simulink model "cpu_von_nuemann"  (R2020a)
settings: Solver=VariableStepAuto  StartTime=0.0  StopTime=10.0  RelTol=1e-3
libraries: simulink_extras x402, msbPllFoundation x1
(part 16 of 64)

== system cpu_von_nuemann/CPU/ALU/Subsystem7/Subsystem1/Subsystem4/Subsystem1 ==
  In1 : Inport
  In2 : Inport  Port=2
  In3 : Inport  Port=3
  In4 : Inport  Port=4
  In5 : Inport  Port=5
  In6 : Inport  Port=6
  In7 : Inport  Port=7
  NAND : Logic  Operator=NAND  AllPortsSameDT=off  OutDataTypeStr=boolean
  NAND{1..2,4..6} (5 alike) : Logic  Operator=NAND  Inputs=4  AllPortsSameDT=off  OutDataTypeStr=boolean
  NAND3 : Logic  Operator=NAND  AllPortsSameDT=off  OutDataTypeStr=boolean
  Out1 : Outport
  wires:
  NAND6/1 -> NAND1/4
  In5/1 -> NAND5/3
  NAND3/1 -> NAND4/2, NAND2/2
  In1/1 -> NAND6/2, NAND5/2, NAND3/2, NAND3/1
  In2/1 -> NAND6/1, NAND4/1, NAND/2, NAND/1
  In4/1 -> NAND4/3
  In3/1 -> NAND2/3
  NAND/1 -> NAND5/1, NAND2/1
  NAND1/1 -> Out1/1
  In6/1 -> NAND6/3
  NAND5/1 -> NAND1/3
  NAND4/1 -> NAND1/2
  In7/1 -> NAND2/4, NAND4/4, NAND5/4, NAND6/4
  NAND2/1 -> NAND1/1

== system cpu_von_nuemann/CPU/ALU/Subsystem7/Subsystem1/Subsystem4/Subsystem2 ==
  In1 : Inport
  In2 : Inport  Port=2
  In3 : Inport  Port=3
  In4 : Inport  Port=4
  In5 : Inport  Port=5
  In6 : Inport  Port=6
  In7 : Inport  Port=7
  NAND : Logic  Operator=NAND  AllPortsSameDT=off  OutDataTypeStr=boolean
  NAND{1..2,4..6} (5 alike) : Logic  Operator=NAND  Inputs=4  AllPortsSameDT=off  OutDataTypeStr=boolean
  NAND3 : Logic  Operator=NAND  AllPortsSameDT=off  OutDataTypeStr=boolean
  Out1 : Outport
  wires:
  NAND6/1 -> NAND1/4
  In5/1 -> NAND5/3
  NAND3/1 -> NAND4/2, NAND2/2
  In1/1 -> NAND6/2, NAND5/2, NAND3/2, NAND3/1
  In2/1 -> NAND6/1, NAND4/1, NAND/2, NAND/1
  In4/1 -> NAND4/3
  In3/1 -> NAND2/3
  NAND/1 -> NAND5/1, NAND2/1
  NAND1/1 -> Out1/1
  In6/1 -> NAND6/3
  NAND5/1 -> NAND1/3
  NAND4/1 -> NAND1/2
  In7/1 -> NAND2/4, NAND4/4, NAND5/4, NAND6/4
  NAND2/1 -> NAND1/1

== system cpu_von_nuemann/CPU/ALU/Subsystem7/Subsystem1/Subsystem4/Subsystem3 ==
  In1 : Inport
  In2 : Inport  Port=2
  In3 : Inport  Port=3
  In4 : Inport  Port=4
  In5 : Inport  Port=5
  In6 : Inport  Port=6
  In7 : Inport  Port=7
  NAND : Logic  Operator=NAND  AllPortsSameDT=off  OutDataTypeStr=boolean
  NAND{1..2,4..6} (5 alike) : Logic  Operator=NAND  Inputs=4  AllPortsSameDT=off  OutDataTypeStr=boolean
  NAND3 : Logic  Operator=NAND  AllPortsSameDT=off  OutDataTypeStr=boolean
  Out1 : Outport
  wires:
  NAND6/1 -> NAND1/4
  In5/1 -> NAND5/3
  NAND3/1 -> NAND4/2, NAND2/2
  In1/1 -> NAND6/2, NAND5/2, NAND3/2, NAND3/1
  In2/1 -> NAND6/1, NAND4/1, NAND/2, NAND/1
  In4/1 -> NAND4/3
  In3/1 -> NAND2/3
  NAND/1 -> NAND5/1, NAND2/1
  NAND1/1 -> Out1/1
  In6/1 -> NAND6/3
  NAND5/1 -> NAND1/3
  NAND4/1 -> NAND1/2
  In7/1 -> NAND2/4, NAND4/4, NAND5/4, NAND6/4
  NAND2/1 -> NAND1/1

== system cpu_von_nuemann/CPU/ALU/Subsystem7/Subsystem1/Subsystem4/Subsystem4 ==
  In1 : Inport
  In2 : Inport  Port=2
  In3 : Inport  Port=3
  In4 : Inport  Port=4
  In5 : Inport  Port=5
  In6 : Inport  Port=6
  In7 : Inport  Port=7
  NAND : Logic  Operator=NAND  AllPortsSameDT=off  OutDataTypeStr=boolean
  NAND{1..2,4..6} (5 alike) : Logic  Operator=NAND  Inputs=4  AllPortsSameDT=off  OutDataTypeStr=boolean
  NAND3 : Logic  Operator=NAND  AllPortsSameDT=off  OutDataTypeStr=boolean
  Out1 : Outport
  wires:
  NAND6/1 -> NAND1/4
  In5/1 -> NAND5/3
  NAND3/1 -> NAND4/2, NAND2/2
  In1/1 -> NAND6/2, NAND5/2, NAND3/2, NAND3/1
  In2/1 -> NAND6/1, NAND4/1, NAND/2, NAND/1
  In4/1 -> NAND4/3
  In3/1 -> NAND2/3
  NAND/1 -> NAND5/1, NAND2/1
  NAND1/1 -> Out1/1
  In6/1 -> NAND6/3
  NAND5/1 -> NAND1/3
  NAND4/1 -> NAND1/2
  In7/1 -> NAND2/4, NAND4/4, NAND5/4, NAND6/4
  NAND2/1 -> NAND1/1

== system cpu_von_nuemann/CPU/ALU/Subsystem7/Subsystem1/Subsystem4/Subsystem5 ==
  In1 : Inport
  In2 : Inport  Port=2
  In3 : Inport  Port=3
  In4 : Inport  Port=4
  In5 : Inport  Port=5
  In6 : Inport  Port=6
  In7 : Inport  Port=7
  NAND : Logic  Operator=NAND  AllPortsSameDT=off  OutDataTypeStr=boolean
  NAND{1..2,4..6} (5 alike) : Logic  Operator=NAND  Inputs=4  AllPortsSameDT=off  OutDataTypeStr=boolean
  NAND3 : Logic  Operator=NAND  AllPortsSameDT=off  OutDataTypeStr=boolean
  Out1 : Outport
  wires:
  NAND6/1 -> NAND1/4
  In5/1 -> NAND5/3
  NAND3/1 -> NAND4/2, NAND2/2
  In1/1 -> NAND6/2, NAND5/2, NAND3/2, NAND3/1
  In2/1 -> NAND6/1, NAND4/1, NAND/2, NAND/1
  In4/1 -> NAND4/3
  In3/1 -> NAND2/3
  NAND/1 -> NAND5/1, NAND2/1
  NAND1/1 -> Out1/1
  In6/1 -> NAND6/3
  NAND5/1 -> NAND1/3
  NAND4/1 -> NAND1/2
  In7/1 -> NAND2/4, NAND4/4, NAND5/4, NAND6/4
  NAND2/1 -> NAND1/1

== system cpu_von_nuemann/CPU/ALU/Subsystem7/Subsystem1/Subsystem4/Subsystem6 ==
  In1 : Inport
  In2 : Inport  Port=2
  In3 : Inport  Port=3
  In4 : Inport  Port=4
  In5 : Inport  Port=5
  In6 : Inport  Port=6
  In7 : Inport  Port=7
  NAND : Logic  Operator=NAND  AllPortsSameDT=off  OutDataTypeStr=boolean
  NAND{1..2,4..6} (5 alike) : Logic  Operator=NAND  Inputs=4  AllPortsSameDT=off  OutDataTypeStr=boolean
  NAND3 : Logic  Operator=NAND  AllPortsSameDT=off  OutDataTypeStr=boolean
  Out1 : Outport
  wires:
  NAND6/1 -> NAND1/4
  In5/1 -> NAND5/3
  NAND3/1 -> NAND4/2, NAND2/2
  In1/1 -> NAND6/2, NAND5/2, NAND3/2, NAND3/1
  In2/1 -> NAND6/1, NAND4/1, NAND/2, NAND/1
  In4/1 -> NAND4/3
  In3/1 -> NAND2/3
  NAND/1 -> NAND5/1, NAND2/1
  NAND1/1 -> Out1/1
  In6/1 -> NAND6/3
  NAND5/1 -> NAND1/3
  NAND4/1 -> NAND1/2
  In7/1 -> NAND2/4, NAND4/4, NAND5/4, NAND6/4
  NAND2/1 -> NAND1/1

== system cpu_von_nuemann/CPU/ALU/Subsystem7/Subsystem1/Subsystem4/Subsystem7 ==
  In1 : Inport
  In2 : Inport  Port=2
  In3 : Inport  Port=3
  In4 : Inport  Port=4
  In5 : Inport  Port=5
  In6 : Inport  Port=6
  In7 : Inport  Port=7
  NAND : Logic  Operator=NAND  AllPortsSameDT=off  OutDataTypeStr=boolean
  NAND{1..2,4..6} (5 alike) : Logic  Operator=NAND  Inputs=4  AllPortsSameDT=off  OutDataTypeStr=boolean
  NAND3 : Logic  Operator=NAND  AllPortsSameDT=off  OutDataTypeStr=boolean
  Out1 : Outport
  wires:
  NAND6/1 -> NAND1/4
  In5/1 -> NAND5/3
  NAND3/1 -> NAND4/2, NAND2/2
  In1/1 -> NAND6/2, NAND5/2, NAND3/2, NAND3/1
  In2/1 -> NAND6/1, NAND4/1, NAND/2, NAND/1
  In4/1 -> NAND4/3
  In3/1 -> NAND2/3
  NAND/1 -> NAND5/1, NAND2/1
  NAND1/1 -> Out1/1
  In6/1 -> NAND6/3
  NAND5/1 -> NAND1/3
  NAND4/1 -> NAND1/2
  In7/1 -> NAND2/4, NAND4/4, NAND5/4, NAND6/4
  NAND2/1 -> NAND1/1

== system cpu_von_nuemann/CPU/ALU/Subsystem7/Subsystem1/Subsystem5/Subsystem ==
  In1 : Inport
  In2 : Inport  Port=2
  In3 : Inport  Port=3
  In4 : Inport  Port=4
  In5 : Inport  Port=5
  In6 : Inport  Port=6
  In7 : Inport  Port=7
  NAND : Logic  Operator=NAND  AllPortsSameDT=off  OutDataTypeStr=boolean
  NAND{1..2,4..6} (5 alike) : Logic  Operator=NAND  Inputs=4  AllPortsSameDT=off  OutDataTypeStr=boolean
  NAND3 : Logic  Operator=NAND  AllPortsSameDT=off  OutDataTypeStr=boolean
  Out1 : Outport
  wires:
  NAND6/1 -> NAND1/4
  In5/1 -> NAND5/3
  NAND3/1 -> NAND4/2, NAND2/2
  In1/1 -> NAND6/2, NAND5/2, NAND3/2, NAND3/1
  In2/1 -> NAND6/1, NAND4/1, NAND/2, NAND/1
  In4/1 -> NAND4/3
  In3/1 -> NAND2/3
  NAND/1 -> NAND5/1, NAND2/1
  NAND1/1 -> Out1/1
  In6/1 -> NAND6/3
  NAND5/1 -> NAND1/3
  NAND4/1 -> NAND1/2
  In7/1 -> NAND2/4, NAND4/4, NAND5/4, NAND6/4
  NAND2/1 -> NAND1/1

== system cpu_von_nuemann/CPU/ALU/Subsystem7/Subsystem1/Subsystem5/Subsystem1 ==
  In1 : Inport
  In2 : Inport  Port=2
  In3 : Inport  Port=3
  In4 : Inport  Port=4
  In5 : Inport  Port=5
  In6 : Inport  Port=6
  In7 : Inport  Port=7
  NAND : Logic  Operator=NAND  AllPortsSameDT=off  OutDataTypeStr=boolean
  NAND{1..2,4..6} (5 alike) : Logic  Operator=NAND  Inputs=4  AllPortsSameDT=off  OutDataTypeStr=boolean
  NAND3 : Logic  Operator=NAND  AllPortsSameDT=off  OutDataTypeStr=boolean
  Out1 : Outport
  wires:
  NAND6/1 -> NAND1/4
  In5/1 -> NAND5/3
  NAND3/1 -> NAND4/2, NAND2/2
  In1/1 -> NAND6/2, NAND5/2, NAND3/2, NAND3/1
  In2/1 -> NAND6/1, NAND4/1, NAND/2, NAND/1
  In4/1 -> NAND4/3
  In3/1 -> NAND2/3
  NAND/1 -> NAND5/1, NAND2/1
  NAND1/1 -> Out1/1
  In6/1 -> NAND6/3
  NAND5/1 -> NAND1/3
  NAND4/1 -> NAND1/2
  In7/1 -> NAND2/4, NAND4/4, NAND5/4, NAND6/4
  NAND2/1 -> NAND1/1

== system cpu_von_nuemann/CPU/ALU/Subsystem7/Subsystem1/Subsystem5/Subsystem2 ==
  In1 : Inport
  In2 : Inport  Port=2
  In3 : Inport  Port=3
  In4 : Inport  Port=4
  In5 : Inport  Port=5
  In6 : Inport  Port=6
  In7 : Inport  Port=7
  NAND : Logic  Operator=NAND  AllPortsSameDT=off  OutDataTypeStr=boolean
  NAND{1..2,4..6} (5 alike) : Logic  Operator=NAND  Inputs=4  AllPortsSameDT=off  OutDataTypeStr=boolean
  NAND3 : Logic  Operator=NAND  AllPortsSameDT=off  OutDataTypeStr=boolean
  Out1 : Outport
  wires:
  NAND6/1 -> NAND1/4
  In5/1 -> NAND5/3
  NAND3/1 -> NAND4/2, NAND2/2
  In1/1 -> NAND6/2, NAND5/2, NAND3/2, NAND3/1
  In2/1 -> NAND6/1, NAND4/1, NAND/2, NAND/1
  In4/1 -> NAND4/3
  In3/1 -> NAND2/3
  NAND/1 -> NAND5/1, NAND2/1
  NAND1/1 -> Out1/1
  In6/1 -> NAND6/3
  NAND5/1 -> NAND1/3
  NAND4/1 -> NAND1/2
  In7/1 -> NAND2/4, NAND4/4, NAND5/4, NAND6/4
  NAND2/1 -> NAND1/1

== system cpu_von_nuemann/CPU/ALU/Subsystem7/Subsystem1/Subsystem5/Subsystem3 ==
  In1 : Inport
  In2 : Inport  Port=2
  In3 : Inport  Port=3
  In4 : Inport  Port=4
  In5 : Inport  Port=5
  In6 : Inport  Port=6
  In7 : Inport  Port=7
  NAND : Logic  Operator=NAND  AllPortsSameDT=off  OutDataTypeStr=boolean
  NAND{1..2,4..6} (5 alike) : Logic  Operator=NAND  Inputs=4  AllPortsSameDT=off  OutDataTypeStr=boolean
  NAND3 : Logic  Operator=NAND  AllPortsSameDT=off  OutDataTypeStr=boolean
  Out1 : Outport
  wires:
  NAND6/1 -> NAND1/4
  In5/1 -> NAND5/3
  NAND3/1 -> NAND4/2, NAND2/2
  In1/1 -> NAND6/2, NAND5/2, NAND3/2, NAND3/1
  In2/1 -> NAND6/1, NAND4/1, NAND/2, NAND/1
  In4/1 -> NAND4/3
  In3/1 -> NAND2/3
  NAND/1 -> NAND5/1, NAND2/1
  NAND1/1 -> Out1/1
  In6/1 -> NAND6/3
  NAND5/1 -> NAND1/3
  NAND4/1 -> NAND1/2
  In7/1 -> NAND2/4, NAND4/4, NAND5/4, NAND6/4
  NAND2/1 -> NAND1/1

== system cpu_von_nuemann/CPU/ALU/Subsystem7/Subsystem1/Subsystem5/Subsystem4 ==
  In1 : Inport
  In2 : Inport  Port=2
  In3 : Inport  Port=3
  In4 : Inport  Port=4
  In5 : Inport  Port=5
  In6 : Inport  Port=6
  In7 : Inport  Port=7
  NAND : Logic  Operator=NAND  AllPortsSameDT=off  OutDataTypeStr=boolean
  NAND{1..2,4..6} (5 alike) : Logic  Operator=NAND  Inputs=4  AllPortsSameDT=off  OutDataTypeStr=boolean
  NAND3 : Logic  Operator=NAND  AllPortsSameDT=off  OutDataTypeStr=boolean
  Out1 : Outport
  wires:
  NAND6/1 -> NAND1/4
  In5/1 -> NAND5/3
  NAND3/1 -> NAND4/2, NAND2/2
  In1/1 -> NAND6/2, NAND5/2, NAND3/2, NAND3/1
  In2/1 -> NAND6/1, NAND4/1, NAND/2, NAND/1
  In4/1 -> NAND4/3
  In3/1 -> NAND2/3
  NAND/1 -> NAND5/1, NAND2/1
  NAND1/1 -> Out1/1
  In6/1 -> NAND6/3
  NAND5/1 -> NAND1/3
  NAND4/1 -> NAND1/2
  In7/1 -> NAND2/4, NAND4/4, NAND5/4, NAND6/4
  NAND2/1 -> NAND1/1

== system cpu_von_nuemann/CPU/ALU/Subsystem7/Subsystem1/Subsystem5/Subsystem5 ==
  In1 : Inport
  In2 : Inport  Port=2
  In3 : Inport  Port=3
  In4 : Inport  Port=4
  In5 : Inport  Port=5
  In6 : Inport  Port=6
  In7 : Inport  Port=7
  NAND : Logic  Operator=NAND  AllPortsSameDT=off  OutDataTypeStr=boolean
  NAND{1..2,4..6} (5 alike) : Logic  Operator=NAND  Inputs=4  AllPortsSameDT=off  OutDataTypeStr=boolean
  NAND3 : Logic  Operator=NAND  AllPortsSameDT=off  OutDataTypeStr=boolean
  Out1 : Outport
  wires:
  NAND6/1 -> NAND1/4
  In5/1 -> NAND5/3
  NAND3/1 -> NAND4/2, NAND2/2
  In1/1 -> NAND6/2, NAND5/2, NAND3/2, NAND3/1
  In2/1 -> NAND6/1, NAND4/1, NAND/2, NAND/1
  In4/1 -> NAND4/3
  In3/1 -> NAND2/3
  NAND/1 -> NAND5/1, NAND2/1
  NAND1/1 -> Out1/1
  In6/1 -> NAND6/3
  NAND5/1 -> NAND1/3
  NAND4/1 -> NAND1/2
  In7/1 -> NAND2/4, NAND4/4, NAND5/4, NAND6/4
  NAND2/1 -> NAND1/1

== system cpu_von_nuemann/CPU/ALU/Subsystem7/Subsystem1/Subsystem5/Subsystem6 ==
  In1 : Inport
  In2 : Inport  Port=2
  In3 : Inport  Port=3
  In4 : Inport  Port=4
  In5 : Inport  Port=5
  In6 : Inport  Port=6
  In7 : Inport  Port=7
  NAND : Logic  Operator=NAND  AllPortsSameDT=off  OutDataTypeStr=boolean
  NAND{1..2,4..6} (5 alike) : Logic  Operator=NAND  Inputs=4  AllPortsSameDT=off  OutDataTypeStr=boolean
  NAND3 : Logic  Operator=NAND  AllPortsSameDT=off  OutDataTypeStr=boolean
  Out1 : Outport
  wires:
  NAND6/1 -> NAND1/4
  In5/1 -> NAND5/3
  NAND3/1 -> NAND4/2, NAND2/2
  In1/1 -> NAND6/2, NAND5/2, NAND3/2, NAND3/1
  In2/1 -> NAND6/1, NAND4/1, NAND/2, NAND/1
  In4/1 -> NAND4/3
  In3/1 -> NAND2/3
  NAND/1 -> NAND5/1, NAND2/1
  NAND1/1 -> Out1/1
  In6/1 -> NAND6/3
  NAND5/1 -> NAND1/3
  NAND4/1 -> NAND1/2
  In7/1 -> NAND2/4, NAND4/4, NAND5/4, NAND6/4
  NAND2/1 -> NAND1/1

== system cpu_von_nuemann/CPU/ALU/Subsystem7/Subsystem1/Subsystem5/Subsystem7 ==
  In1 : Inport
  In2 : Inport  Port=2
  In3 : Inport  Port=3
  In4 : Inport  Port=4
  In5 : Inport  Port=5
  In6 : Inport  Port=6
  In7 : Inport  Port=7
  NAND : Logic  Operator=NAND  AllPortsSameDT=off  OutDataTypeStr=boolean
  NAND{1..2,4..6} (5 alike) : Logic  Operator=NAND  Inputs=4  AllPortsSameDT=off  OutDataTypeStr=boolean
  NAND3 : Logic  Operator=NAND  AllPortsSameDT=off  OutDataTypeStr=boolean
  Out1 : Outport
  wires:
  NAND6/1 -> NAND1/4
  In5/1 -> NAND5/3
  NAND3/1 -> NAND4/2, NAND2/2
  In1/1 -> NAND6/2, NAND5/2, NAND3/2, NAND3/1
  In2/1 -> NAND6/1, NAND4/1, NAND/2, NAND/1
  In4/1 -> NAND4/3
  In3/1 -> NAND2/3
  NAND/1 -> NAND5/1, NAND2/1
  NAND1/1 -> Out1/1
  In6/1 -> NAND6/3
  NAND5/1 -> NAND1/3
  NAND4/1 -> NAND1/2
  In7/1 -> NAND2/4, NAND4/4, NAND5/4, NAND6/4
  NAND2/1 -> NAND1/1

== system cpu_von_nuemann/CPU/ALU/Subsystem7/Subsystem2/Subsystem1/Subsystem ==
  In1 : Inport
  In2 : Inport  Port=2
  In3 : Inport  Port=3
  In4 : Inport  Port=4
  In5 : Inport  Port=5
  In6 : Inport  Port=6
  In7 : Inport  Port=7
  NAND : Logic  Operator=NAND  AllPortsSameDT=off  OutDataTypeStr=boolean
  NAND{1..2,4..6} (5 alike) : Logic  Operator=NAND  Inputs=4  AllPortsSameDT=off  OutDataTypeStr=boolean
  NAND3 : Logic  Operator=NAND  AllPortsSameDT=off  OutDataTypeStr=boolean
  Out1 : Outport
  wires:
  NAND6/1 -> NAND1/4
  In5/1 -> NAND5/3
  NAND3/1 -> NAND4/2, NAND2/2
  In1/1 -> NAND6/2, NAND5/2, NAND3/2, NAND3/1
  In2/1 -> NAND6/1, NAND4/1, NAND/2, NAND/1
  In4/1 -> NAND4/3
  In3/1 -> NAND2/3
  NAND/1 -> NAND5/1, NAND2/1
  NAND1/1 -> Out1/1
  In6/1 -> NAND6/3
  NAND5/1 -> NAND1/3
  NAND4/1 -> NAND1/2
  In7/1 -> NAND2/4, NAND4/4, NAND5/4, NAND6/4
  NAND2/1 -> NAND1/1

== system cpu_von_nuemann/CPU/ALU/Subsystem7/Subsystem2/Subsystem1/Subsystem1 ==
  In1 : Inport
  In2 : Inport  Port=2
  In3 : Inport  Port=3
  In4 : Inport  Port=4
  In5 : Inport  Port=5
  In6 : Inport  Port=6
  In7 : Inport  Port=7
  NAND : Logic  Operator=NAND  AllPortsSameDT=off  OutDataTypeStr=boolean
  NAND{1..2,4..6} (5 alike) : Logic  Operator=NAND  Inputs=4  AllPortsSameDT=off  OutDataTypeStr=boolean
  NAND3 : Logic  Operator=NAND  AllPortsSameDT=off  OutDataTypeStr=boolean
  Out1 : Outport
  wires:
  NAND6/1 -> NAND1/4
  In5/1 -> NAND5/3
  NAND3/1 -> NAND4/2, NAND2/2
  In1/1 -> NAND6/2, NAND5/2, NAND3/2, NAND3/1
  In2/1 -> NAND6/1, NAND4/1, NAND/2, NAND/1
  In4/1 -> NAND4/3
  In3/1 -> NAND2/3
  NAND/1 -> NAND5/1, NAND2/1
  NAND1/1 -> Out1/1
  In6/1 -> NAND6/3
  NAND5/1 -> NAND1/3
  NAND4/1 -> NAND1/2
  In7/1 -> NAND2/4, NAND4/4, NAND5/4, NAND6/4
  NAND2/1 -> NAND1/1

== system cpu_von_nuemann/CPU/ALU/Subsystem7/Subsystem2/Subsystem1/Subsystem2 ==
  In1 : Inport
  In2 : Inport  Port=2
  In3 : Inport  Port=3
  In4 : Inport  Port=4
  In5 : Inport  Port=5
  In6 : Inport  Port=6
  In7 : Inport  Port=7
  NAND : Logic  Operator=NAND  AllPortsSameDT=off  OutDataTypeStr=boolean
  NAND{1..2,4..6} (5 alike) : Logic  Operator=NAND  Inputs=4  AllPortsSameDT=off  OutDataTypeStr=boolean
  NAND3 : Logic  Operator=NAND  AllPortsSameDT=off  OutDataTypeStr=boolean
  Out1 : Outport
  wires:
  NAND6/1 -> NAND1/4
  In5/1 -> NAND5/3
  NAND3/1 -> NAND4/2, NAND2/2
  In1/1 -> NAND6/2, NAND5/2, NAND3/2, NAND3/1
  In2/1 -> NAND6/1, NAND4/1, NAND/2, NAND/1
  In4/1 -> NAND4/3
  In3/1 -> NAND2/3
  NAND/1 -> NAND5/1, NAND2/1
  NAND1/1 -> Out1/1
  In6/1 -> NAND6/3
  NAND5/1 -> NAND1/3
  NAND4/1 -> NAND1/2
  In7/1 -> NAND2/4, NAND4/4, NAND5/4, NAND6/4
  NAND2/1 -> NAND1/1

== system cpu_von_nuemann/CPU/ALU/Subsystem7/Subsystem2/Subsystem1/Subsystem3 ==
  In1 : Inport
  In2 : Inport  Port=2
  In3 : Inport  Port=3
  In4 : Inport  Port=4
  In5 : Inport  Port=5
  In6 : Inport  Port=6
  In7 : Inport  Port=7
  NAND : Logic  Operator=NAND  AllPortsSameDT=off  OutDataTypeStr=boolean
  NAND{1..2,4..6} (5 alike) : Logic  Operator=NAND  Inputs=4  AllPortsSameDT=off  OutDataTypeStr=boolean
  NAND3 : Logic  Operator=NAND  AllPortsSameDT=off  OutDataTypeStr=boolean
  Out1 : Outport
  wires:
  NAND6/1 -> NAND1/4
  In5/1 -> NAND5/3
  NAND3/1 -> NAND4/2, NAND2/2
  In1/1 -> NAND6/2, NAND5/2, NAND3/2, NAND3/1
  In2/1 -> NAND6/1, NAND4/1, NAND/2, NAND/1
  In4/1 -> NAND4/3
  In3/1 -> NAND2/3
  NAND/1 -> NAND5/1, NAND2/1
  NAND1/1 -> Out1/1
  In6/1 -> NAND6/3
  NAND5/1 -> NAND1/3
  NAND4/1 -> NAND1/2
  In7/1 -> NAND2/4, NAND4/4, NAND5/4, NAND6/4
  NAND2/1 -> NAND1/1

== system cpu_von_nuemann/CPU/ALU/Subsystem7/Subsystem2/Subsystem1/Subsystem4 ==
  In1 : Inport
  In2 : Inport  Port=2
  In3 : Inport  Port=3
  In4 : Inport  Port=4
  In5 : Inport  Port=5
  In6 : Inport  Port=6
  In7 : Inport  Port=7
  NAND : Logic  Operator=NAND  AllPortsSameDT=off  OutDataTypeStr=boolean
  NAND{1..2,4..6} (5 alike) : Logic  Operator=NAND  Inputs=4  AllPortsSameDT=off  OutDataTypeStr=boolean
  NAND3 : Logic  Operator=NAND  AllPortsSameDT=off  OutDataTypeStr=boolean
  Out1 : Outport
  wires:
  NAND6/1 -> NAND1/4
  In5/1 -> NAND5/3
  NAND3/1 -> NAND4/2, NAND2/2
  In1/1 -> NAND6/2, NAND5/2, NAND3/2, NAND3/1
  In2/1 -> NAND6/1, NAND4/1, NAND/2, NAND/1
  In4/1 -> NAND4/3
  In3/1 -> NAND2/3
  NAND/1 -> NAND5/1, NAND2/1
  NAND1/1 -> Out1/1
  In6/1 -> NAND6/3
  NAND5/1 -> NAND1/3
  NAND4/1 -> NAND1/2
  In7/1 -> NAND2/4, NAND4/4, NAND5/4, NAND6/4
  NAND2/1 -> NAND1/1

== system cpu_von_nuemann/CPU/ALU/Subsystem7/Subsystem2/Subsystem1/Subsystem5 ==
  In1 : Inport
  In2 : Inport  Port=2
  In3 : Inport  Port=3
  In4 : Inport  Port=4
  In5 : Inport  Port=5
  In6 : Inport  Port=6
  In7 : Inport  Port=7
  NAND : Logic  Operator=NAND  AllPortsSameDT=off  OutDataTypeStr=boolean
  NAND{1..2,4..6} (5 alike) : Logic  Operator=NAND  Inputs=4  AllPortsSameDT=off  OutDataTypeStr=boolean
  NAND3 : Logic  Operator=NAND  AllPortsSameDT=off  OutDataTypeStr=boolean
  Out1 : Outport
  wires:
  NAND6/1 -> NAND1/4
  In5/1 -> NAND5/3
  NAND3/1 -> NAND4/2, NAND2/2
  In1/1 -> NAND6/2, NAND5/2, NAND3/2, NAND3/1
  In2/1 -> NAND6/1, NAND4/1, NAND/2, NAND/1
  In4/1 -> NAND4/3
  In3/1 -> NAND2/3
  NAND/1 -> NAND5/1, NAND2/1
  NAND1/1 -> Out1/1
  In6/1 -> NAND6/3
  NAND5/1 -> NAND1/3
  NAND4/1 -> NAND1/2
  In7/1 -> NAND2/4, NAND4/4, NAND5/4, NAND6/4
  NAND2/1 -> NAND1/1

== system cpu_von_nuemann/CPU/ALU/Subsystem7/Subsystem2/Subsystem1/Subsystem6 ==
  In1 : Inport
  In2 : Inport  Port=2
  In3 : Inport  Port=3
  In4 : Inport  Port=4
  In5 : Inport  Port=5
  In6 : Inport  Port=6
  In7 : Inport  Port=7
  NAND : Logic  Operator=NAND  AllPortsSameDT=off  OutDataTypeStr=boolean
  NAND{1..2,4..6} (5 alike) : Logic  Operator=NAND  Inputs=4  AllPortsSameDT=off  OutDataTypeStr=boolean
  NAND3 : Logic  Operator=NAND  AllPortsSameDT=off  OutDataTypeStr=boolean
  Out1 : Outport
  wires:
  NAND6/1 -> NAND1/4
  In5/1 -> NAND5/3
  NAND3/1 -> NAND4/2, NAND2/2
  In1/1 -> NAND6/2, NAND5/2, NAND3/2, NAND3/1
  In2/1 -> NAND6/1, NAND4/1, NAND/2, NAND/1
  In4/1 -> NAND4/3
  In3/1 -> NAND2/3
  NAND/1 -> NAND5/1, NAND2/1
  NAND1/1 -> Out1/1
  In6/1 -> NAND6/3
  NAND5/1 -> NAND1/3
  NAND4/1 -> NAND1/2
  In7/1 -> NAND2/4, NAND4/4, NAND5/4, NAND6/4
  NAND2/1 -> NAND1/1

== system cpu_von_nuemann/CPU/ALU/Subsystem7/Subsystem2/Subsystem1/Subsystem7 ==
  In1 : Inport
  In2 : Inport  Port=2
  In3 : Inport  Port=3
  In4 : Inport  Port=4
  In5 : Inport  Port=5
  In6 : Inport  Port=6
  In7 : Inport  Port=7
  NAND : Logic  Operator=NAND  AllPortsSameDT=off  OutDataTypeStr=boolean
  NAND{1..2,4..6} (5 alike) : Logic  Operator=NAND  Inputs=4  AllPortsSameDT=off  OutDataTypeStr=boolean
  NAND3 : Logic  Operator=NAND  AllPortsSameDT=off  OutDataTypeStr=boolean
  Out1 : Outport
  wires:
  NAND6/1 -> NAND1/4
  In5/1 -> NAND5/3
  NAND3/1 -> NAND4/2, NAND2/2
  In1/1 -> NAND6/2, NAND5/2, NAND3/2, NAND3/1
  In2/1 -> NAND6/1, NAND4/1, NAND/2, NAND/1
  In4/1 -> NAND4/3
  In3/1 -> NAND2/3
  NAND/1 -> NAND5/1, NAND2/1
  NAND1/1 -> Out1/1
  In6/1 -> NAND6/3
  NAND5/1 -> NAND1/3
  NAND4/1 -> NAND1/2
  In7/1 -> NAND2/4, NAND4/4, NAND5/4, NAND6/4
  NAND2/1 -> NAND1/1

== system cpu_von_nuemann/CPU/ALU/Subsystem7/Subsystem2/Subsystem2/Subsystem ==
  In1 : Inport
  In2 : Inport  Port=2
  In3 : Inport  Port=3
  In4 : Inport  Port=4
  In5 : Inport  Port=5
  In6 : Inport  Port=6
  In7 : Inport  Port=7
  NAND : Logic  Operator=NAND  AllPortsSameDT=off  OutDataTypeStr=boolean
  NAND{1..2,4..6} (5 alike) : Logic  Operator=NAND  Inputs=4  AllPortsSameDT=off  OutDataTypeStr=boolean
  NAND3 : Logic  Operator=NAND  AllPortsSameDT=off  OutDataTypeStr=boolean
  Out1 : Outport
  wires:
  NAND6/1 -> NAND1/4
  In5/1 -> NAND5/3
  NAND3/1 -> NAND4/2, NAND2/2
  In1/1 -> NAND6/2, NAND5/2, NAND3/2, NAND3/1
  In2/1 -> NAND6/1, NAND4/1, NAND/2, NAND/1
  In4/1 -> NAND4/3
  In3/1 -> NAND2/3
  NAND/1 -> NAND5/1, NAND2/1
  NAND1/1 -> Out1/1
  In6/1 -> NAND6/3
  NAND5/1 -> NAND1/3
  NAND4/1 -> NAND1/2
  In7/1 -> NAND2/4, NAND4/4, NAND5/4, NAND6/4
  NAND2/1 -> NAND1/1

== system cpu_von_nuemann/CPU/ALU/Subsystem7/Subsystem2/Subsystem2/Subsystem1 ==
  In1 : Inport
  In2 : Inport  Port=2
  In3 : Inport  Port=3
  In4 : Inport  Port=4
  In5 : Inport  Port=5
  In6 : Inport  Port=6
  In7 : Inport  Port=7
  NAND : Logic  Operator=NAND  AllPortsSameDT=off  OutDataTypeStr=boolean
  NAND{1..2,4..6} (5 alike) : Logic  Operator=NAND  Inputs=4  AllPortsSameDT=off  OutDataTypeStr=boolean
  NAND3 : Logic  Operator=NAND  AllPortsSameDT=off  OutDataTypeStr=boolean
  Out1 : Outport
  wires:
  NAND6/1 -> NAND1/4
  In5/1 -> NAND5/3
  NAND3/1 -> NAND4/2, NAND2/2
  In1/1 -> NAND6/2, NAND5/2, NAND3/2, NAND3/1
  In2/1 -> NAND6/1, NAND4/1, NAND/2, NAND/1
  In4/1 -> NAND4/3
  In3/1 -> NAND2/3
  NAND/1 -> NAND5/1, NAND2/1
  NAND1/1 -> Out1/1
  In6/1 -> NAND6/3
  NAND5/1 -> NAND1/3
  NAND4/1 -> NAND1/2
  In7/1 -> NAND2/4, NAND4/4, NAND5/4, NAND6/4
  NAND2/1 -> NAND1/1

== system cpu_von_nuemann/CPU/ALU/Subsystem7/Subsystem2/Subsystem2/Subsystem2 ==
  In1 : Inport
  In2 : Inport  Port=2
  In3 : Inport  Port=3
  In4 : Inport  Port=4
  In5 : Inport  Port=5
  In6 : Inport  Port=6
  In7 : Inport  Port=7
  NAND : Logic  Operator=NAND  AllPortsSameDT=off  OutDataTypeStr=boolean
  NAND{1..2,4..6} (5 alike) : Logic  Operator=NAND  Inputs=4  AllPortsSameDT=off  OutDataTypeStr=boolean
  NAND3 : Logic  Operator=NAND  AllPortsSameDT=off  OutDataTypeStr=boolean
  Out1 : Outport
  wires:
  NAND6/1 -> NAND1/4
  In5/1 -> NAND5/3
  NAND3/1 -> NAND4/2, NAND2/2
  In1/1 -> NAND6/2, NAND5/2, NAND3/2, NAND3/1
  In2/1 -> NAND6/1, NAND4/1, NAND/2, NAND/1
  In4/1 -> NAND4/3
  In3/1 -> NAND2/3
  NAND/1 -> NAND5/1, NAND2/1
  NAND1/1 -> Out1/1
  In6/1 -> NAND6/3
  NAND5/1 -> NAND1/3
  NAND4/1 -> NAND1/2
  In7/1 -> NAND2/4, NAND4/4, NAND5/4, NAND6/4
  NAND2/1 -> NAND1/1

== system cpu_von_nuemann/CPU/ALU/Subsystem7/Subsystem2/Subsystem2/Subsystem3 ==
  In1 : Inport
  In2 : Inport  Port=2
  In3 : Inport  Port=3
  In4 : Inport  Port=4
  In5 : Inport  Port=5
  In6 : Inport  Port=6
  In7 : Inport  Port=7
  NAND : Logic  Operator=NAND  AllPortsSameDT=off  OutDataTypeStr=boolean
  NAND{1..2,4..6} (5 alike) : Logic  Operator=NAND  Inputs=4  AllPortsSameDT=off  OutDataTypeStr=boolean
  NAND3 : Logic  Operator=NAND  AllPortsSameDT=off  OutDataTypeStr=boolean
  Out1 : Outport
  wires:
  NAND6/1 -> NAND1/4
  In5/1 -> NAND5/3
  NAND3/1 -> NAND4/2, NAND2/2
  In1/1 -> NAND6/2, NAND5/2, NAND3/2, NAND3/1
  In2/1 -> NAND6/1, NAND4/1, NAND/2, NAND/1
  In4/1 -> NAND4/3
  In3/1 -> NAND2/3
  NAND/1 -> NAND5/1, NAND2/1
  NAND1/1 -> Out1/1
  In6/1 -> NAND6/3
  NAND5/1 -> NAND1/3
  NAND4/1 -> NAND1/2
  In7/1 -> NAND2/4, NAND4/4, NAND5/4, NAND6/4
  NAND2/1 -> NAND1/1

== system cpu_von_nuemann/CPU/ALU/Subsystem7/Subsystem2/Subsystem2/Subsystem4 ==
  In1 : Inport
  In2 : Inport  Port=2
  In3 : Inport  Port=3
  In4 : Inport  Port=4
  In5 : Inport  Port=5
  In6 : Inport  Port=6
  In7 : Inport  Port=7
  NAND : Logic  Operator=NAND  AllPortsSameDT=off  OutDataTypeStr=boolean
  NAND{1..2,4..6} (5 alike) : Logic  Operator=NAND  Inputs=4  AllPortsSameDT=off  OutDataTypeStr=boolean
  NAND3 : Logic  Operator=NAND  AllPortsSameDT=off  OutDataTypeStr=boolean
  Out1 : Outport
  wires:
  NAND6/1 -> NAND1/4
  In5/1 -> NAND5/3
  NAND3/1 -> NAND4/2, NAND2/2
  In1/1 -> NAND6/2, NAND5/2, NAND3/2, NAND3/1
  In2/1 -> NAND6/1, NAND4/1, NAND/2, NAND/1
  In4/1 -> NAND4/3
  In3/1 -> NAND2/3
  NAND/1 -> NAND5/1, NAND2/1
  NAND1/1 -> Out1/1
  In6/1 -> NAND6/3
  NAND5/1 -> NAND1/3
  NAND4/1 -> NAND1/2
  In7/1 -> NAND2/4, NAND4/4, NAND5/4, NAND6/4
  NAND2/1 -> NAND1/1

== system cpu_von_nuemann/CPU/ALU/Subsystem7/Subsystem2/Subsystem2/Subsystem5 ==
  In1 : Inport
  In2 : Inport  Port=2
  In3 : Inport  Port=3
  In4 : Inport  Port=4
  In5 : Inport  Port=5
  In6 : Inport  Port=6
  In7 : Inport  Port=7
  NAND : Logic  Operator=NAND  AllPortsSameDT=off  OutDataTypeStr=boolean
  NAND{1..2,4..6} (5 alike) : Logic  Operator=NAND  Inputs=4  AllPortsSameDT=off  OutDataTypeStr=boolean
  NAND3 : Logic  Operator=NAND  AllPortsSameDT=off  OutDataTypeStr=boolean
  Out1 : Outport
  wires:
  NAND6/1 -> NAND1/4
  In5/1 -> NAND5/3
  NAND3/1 -> NAND4/2, NAND2/2
  In1/1 -> NAND6/2, NAND5/2, NAND3/2, NAND3/1
  In2/1 -> NAND6/1, NAND4/1, NAND/2, NAND/1
  In4/1 -> NAND4/3
  In3/1 -> NAND2/3
  NAND/1 -> NAND5/1, NAND2/1
  NAND1/1 -> Out1/1
  In6/1 -> NAND6/3
  NAND5/1 -> NAND1/3
  NAND4/1 -> NAND1/2
  In7/1 -> NAND2/4, NAND4/4, NAND5/4, NAND6/4
  NAND2/1 -> NAND1/1

== system cpu_von_nuemann/CPU/ALU/Subsystem7/Subsystem2/Subsystem2/Subsystem6 ==
  In1 : Inport
  In2 : Inport  Port=2
  In3 : Inport  Port=3
  In4 : Inport  Port=4
  In5 : Inport  Port=5
  In6 : Inport  Port=6
  In7 : Inport  Port=7
  NAND : Logic  Operator=NAND  AllPortsSameDT=off  OutDataTypeStr=boolean
  NAND{1..2,4..6} (5 alike) : Logic  Operator=NAND  Inputs=4  AllPortsSameDT=off  OutDataTypeStr=boolean
  NAND3 : Logic  Operator=NAND  AllPortsSameDT=off  OutDataTypeStr=boolean
  Out1 : Outport
  wires:
  NAND6/1 -> NAND1/4
  In5/1 -> NAND5/3
  NAND3/1 -> NAND4/2, NAND2/2
  In1/1 -> NAND6/2, NAND5/2, NAND3/2, NAND3/1
  In2/1 -> NAND6/1, NAND4/1, NAND/2, NAND/1
  In4/1 -> NAND4/3
  In3/1 -> NAND2/3
  NAND/1 -> NAND5/1, NAND2/1
  NAND1/1 -> Out1/1
  In6/1 -> NAND6/3
  NAND5/1 -> NAND1/3
  NAND4/1 -> NAND1/2
  In7/1 -> NAND2/4, NAND4/4, NAND5/4, NAND6/4
  NAND2/1 -> NAND1/1

== system cpu_von_nuemann/CPU/ALU/Subsystem7/Subsystem2/Subsystem2/Subsystem7 ==
  In1 : Inport
  In2 : Inport  Port=2
  In3 : Inport  Port=3
  In4 : Inport  Port=4
  In5 : Inport  Port=5
  In6 : Inport  Port=6
  In7 : Inport  Port=7
  NAND : Logic  Operator=NAND  AllPortsSameDT=off  OutDataTypeStr=boolean
  NAND{1..2,4..6} (5 alike) : Logic  Operator=NAND  Inputs=4  AllPortsSameDT=off  OutDataTypeStr=boolean
  NAND3 : Logic  Operator=NAND  AllPortsSameDT=off  OutDataTypeStr=boolean
  Out1 : Outport
  wires:
  NAND6/1 -> NAND1/4
  In5/1 -> NAND5/3
  NAND3/1 -> NAND4/2, NAND2/2
  In1/1 -> NAND6/2, NAND5/2, NAND3/2, NAND3/1
  In2/1 -> NAND6/1, NAND4/1, NAND/2, NAND/1
  In4/1 -> NAND4/3
  In3/1 -> NAND2/3
  NAND/1 -> NAND5/1, NAND2/1
  NAND1/1 -> Out1/1
  In6/1 -> NAND6/3
  NAND5/1 -> NAND1/3
  NAND4/1 -> NAND1/2
  In7/1 -> NAND2/4, NAND4/4, NAND5/4, NAND6/4
  NAND2/1 -> NAND1/1

== system cpu_von_nuemann/CPU/ALU/Subsystem7/Subsystem2/Subsystem3/Subsystem ==
  In1 : Inport
  In2 : Inport  Port=2
  In3 : Inport  Port=3
  In4 : Inport  Port=4
  In5 : Inport  Port=5
  In6 : Inport  Port=6
  In7 : Inport  Port=7
  NAND : Logic  Operator=NAND  AllPortsSameDT=off  OutDataTypeStr=boolean
  NAND{1..2,4..6} (5 alike) : Logic  Operator=NAND  Inputs=4  AllPortsSameDT=off  OutDataTypeStr=boolean
  NAND3 : Logic  Operator=NAND  AllPortsSameDT=off  OutDataTypeStr=boolean
  Out1 : Outport
  wires:
  NAND6/1 -> NAND1/4
  In5/1 -> NAND5/3
  NAND3/1 -> NAND4/2, NAND2/2
  In1/1 -> NAND6/2, NAND5/2, NAND3/2, NAND3/1
  In2/1 -> NAND6/1, NAND4/1, NAND/2, NAND/1
  In4/1 -> NAND4/3
  In3/1 -> NAND2/3
  NAND/1 -> NAND5/1, NAND2/1
  NAND1/1 -> Out1/1
  In6/1 -> NAND6/3
  NAND5/1 -> NAND1/3
  NAND4/1 -> NAND1/2
  In7/1 -> NAND2/4, NAND4/4, NAND5/4, NAND6/4
  NAND2/1 -> NAND1/1

== system cpu_von_nuemann/CPU/ALU/Subsystem7/Subsystem2/Subsystem3/Subsystem1 ==
  In1 : Inport
  In2 : Inport  Port=2
  In3 : Inport  Port=3
  In4 : Inport  Port=4
  In5 : Inport  Port=5
  In6 : Inport  Port=6
  In7 : Inport  Port=7
  NAND : Logic  Operator=NAND  AllPortsSameDT=off  OutDataTypeStr=boolean
  NAND{1..2,4..6} (5 alike) : Logic  Operator=NAND  Inputs=4  AllPortsSameDT=off  OutDataTypeStr=boolean
  NAND3 : Logic  Operator=NAND  AllPortsSameDT=off  OutDataTypeStr=boolean
  Out1 : Outport
  wires:
  NAND6/1 -> NAND1/4
  In5/1 -> NAND5/3
  NAND3/1 -> NAND4/2, NAND2/2
  In1/1 -> NAND6/2, NAND5/2, NAND3/2, NAND3/1
  In2/1 -> NAND6/1, NAND4/1, NAND/2, NAND/1
  In4/1 -> NAND4/3
  In3/1 -> NAND2/3
  NAND/1 -> NAND5/1, NAND2/1
  NAND1/1 -> Out1/1
  In6/1 -> NAND6/3
  NAND5/1 -> NAND1/3
  NAND4/1 -> NAND1/2
  In7/1 -> NAND2/4, NAND4/4, NAND5/4, NAND6/4
  NAND2/1 -> NAND1/1

== system cpu_von_nuemann/CPU/ALU/Subsystem7/Subsystem2/Subsystem3/Subsystem2 ==
  In1 : Inport
  In2 : Inport  Port=2
  In3 : Inport  Port=3
  In4 : Inport  Port=4
  In5 : Inport  Port=5
  In6 : Inport  Port=6
  In7 : Inport  Port=7
  NAND : Logic  Operator=NAND  AllPortsSameDT=off  OutDataTypeStr=boolean
  NAND{1..2,4..6} (5 alike) : Logic  Operator=NAND  Inputs=4  AllPortsSameDT=off  OutDataTypeStr=boolean
  NAND3 : Logic  Operator=NAND  AllPortsSameDT=off  OutDataTypeStr=boolean
  Out1 : Outport
  wires:
  NAND6/1 -> NAND1/4
  In5/1 -> NAND5/3
  NAND3/1 -> NAND4/2, NAND2/2
  In1/1 -> NAND6/2, NAND5/2, NAND3/2, NAND3/1
  In2/1 -> NAND6/1, NAND4/1, NAND/2, NAND/1
  In4/1 -> NAND4/3
  In3/1 -> NAND2/3
  NAND/1 -> NAND5/1, NAND2/1
  NAND1/1 -> Out1/1
  In6/1 -> NAND6/3
  NAND5/1 -> NAND1/3
  NAND4/1 -> NAND1/2
  In7/1 -> NAND2/4, NAND4/4, NAND5/4, NAND6/4
  NAND2/1 -> NAND1/1

== system cpu_von_nuemann/CPU/ALU/Subsystem7/Subsystem2/Subsystem3/Subsystem3 ==
  In1 : Inport
  In2 : Inport  Port=2
  In3 : Inport  Port=3
  In4 : Inport  Port=4
  In5 : Inport  Port=5
  In6 : Inport  Port=6
  In7 : Inport  Port=7
  NAND : Logic  Operator=NAND  AllPortsSameDT=off  OutDataTypeStr=boolean
  NAND{1..2,4..6} (5 alike) : Logic  Operator=NAND  Inputs=4  AllPortsSameDT=off  OutDataTypeStr=boolean
  NAND3 : Logic  Operator=NAND  AllPortsSameDT=off  OutDataTypeStr=boolean
  Out1 : Outport
  wires:
  NAND6/1 -> NAND1/4
  In5/1 -> NAND5/3
  NAND3/1 -> NAND4/2, NAND2/2
  In1/1 -> NAND6/2, NAND5/2, NAND3/2, NAND3/1
  In2/1 -> NAND6/1, NAND4/1, NAND/2, NAND/1
  In4/1 -> NAND4/3
  In3/1 -> NAND2/3
  NAND/1 -> NAND5/1, NAND2/1
  NAND1/1 -> Out1/1
  In6/1 -> NAND6/3
  NAND5/1 -> NAND1/3
  NAND4/1 -> NAND1/2
  In7/1 -> NAND2/4, NAND4/4, NAND5/4, NAND6/4
  NAND2/1 -> NAND1/1

== system cpu_von_nuemann/CPU/ALU/Subsystem7/Subsystem2/Subsystem3/Subsystem4 ==
  In1 : Inport
  In2 : Inport  Port=2
  In3 : Inport  Port=3
  In4 : Inport  Port=4
  In5 : Inport  Port=5
  In6 : Inport  Port=6
  In7 : Inport  Port=7
  NAND : Logic  Operator=NAND  AllPortsSameDT=off  OutDataTypeStr=boolean
  NAND{1..2,4..6} (5 alike) : Logic  Operator=NAND  Inputs=4  AllPortsSameDT=off  OutDataTypeStr=boolean
  NAND3 : Logic  Operator=NAND  AllPortsSameDT=off  OutDataTypeStr=boolean
  Out1 : Outport
  wires:
  NAND6/1 -> NAND1/4
  In5/1 -> NAND5/3
  NAND3/1 -> NAND4/2, NAND2/2
  In1/1 -> NAND6/2, NAND5/2, NAND3/2, NAND3/1
  In2/1 -> NAND6/1, NAND4/1, NAND/2, NAND/1
  In4/1 -> NAND4/3
  In3/1 -> NAND2/3
  NAND/1 -> NAND5/1, NAND2/1
  NAND1/1 -> Out1/1
  In6/1 -> NAND6/3
  NAND5/1 -> NAND1/3
  NAND4/1 -> NAND1/2
  In7/1 -> NAND2/4, NAND4/4, NAND5/4, NAND6/4
  NAND2/1 -> NAND1/1

== system cpu_von_nuemann/CPU/ALU/Subsystem7/Subsystem2/Subsystem3/Subsystem5 ==
  In1 : Inport
  In2 : Inport  Port=2
  In3 : Inport  Port=3
  In4 : Inport  Port=4
  In5 : Inport  Port=5
  In6 : Inport  Port=6
  In7 : Inport  Port=7
  NAND : Logic  Operator=NAND  AllPortsSameDT=off  OutDataTypeStr=boolean
  NAND{1..2,4..6} (5 alike) : Logic  Operator=NAND  Inputs=4  AllPortsSameDT=off  OutDataTypeStr=boolean
  NAND3 : Logic  Operator=NAND  AllPortsSameDT=off  OutDataTypeStr=boolean
  Out1 : Outport
  wires:
  NAND6/1 -> NAND1/4
  In5/1 -> NAND5/3
  NAND3/1 -> NAND4/2, NAND2/2
  In1/1 -> NAND6/2, NAND5/2, NAND3/2, NAND3/1
  In2/1 -> NAND6/1, NAND4/1, NAND/2, NAND/1
  In4/1 -> NAND4/3
  In3/1 -> NAND2/3
  NAND/1 -> NAND5/1, NAND2/1
  NAND1/1 -> Out1/1
  In6/1 -> NAND6/3
  NAND5/1 -> NAND1/3
  NAND4/1 -> NAND1/2
  In7/1 -> NAND2/4, NAND4/4, NAND5/4, NAND6/4
  NAND2/1 -> NAND1/1

== system cpu_von_nuemann/CPU/ALU/Subsystem7/Subsystem2/Subsystem3/Subsystem6 ==
  In1 : Inport
  In2 : Inport  Port=2
  In3 : Inport  Port=3
  In4 : Inport  Port=4
  In5 : Inport  Port=5
  In6 : Inport  Port=6
  In7 : Inport  Port=7
  NAND : Logic  Operator=NAND  AllPortsSameDT=off  OutDataTypeStr=boolean
  NAND{1..2,4..6} (5 alike) : Logic  Operator=NAND  Inputs=4  AllPortsSameDT=off  OutDataTypeStr=boolean
  NAND3 : Logic  Operator=NAND  AllPortsSameDT=off  OutDataTypeStr=boolean
  Out1 : Outport
  wires:
  NAND6/1 -> NAND1/4
  In5/1 -> NAND5/3
  NAND3/1 -> NAND4/2, NAND2/2
  In1/1 -> NAND6/2, NAND5/2, NAND3/2, NAND3/1
  In2/1 -> NAND6/1, NAND4/1, NAND/2, NAND/1
  In4/1 -> NAND4/3
  In3/1 -> NAND2/3
  NAND/1 -> NAND5/1, NAND2/1
  NAND1/1 -> Out1/1
  In6/1 -> NAND6/3
  NAND5/1 -> NAND1/3
  NAND4/1 -> NAND1/2
  In7/1 -> NAND2/4, NAND4/4, NAND5/4, NAND6/4
  NAND2/1 -> NAND1/1

== system cpu_von_nuemann/CPU/ALU/Subsystem7/Subsystem2/Subsystem3/Subsystem7 ==
  In1 : Inport
  In2 : Inport  Port=2
  In3 : Inport  Port=3
  In4 : Inport  Port=4
  In5 : Inport  Port=5
  In6 : Inport  Port=6
  In7 : Inport  Port=7
  NAND : Logic  Operator=NAND  AllPortsSameDT=off  OutDataTypeStr=boolean
  NAND{1..2,4..6} (5 alike) : Logic  Operator=NAND  Inputs=4  AllPortsSameDT=off  OutDataTypeStr=boolean
  NAND3 : Logic  Operator=NAND  AllPortsSameDT=off  OutDataTypeStr=boolean
  Out1 : Outport
  wires:
  NAND6/1 -> NAND1/4
  In5/1 -> NAND5/3
  NAND3/1 -> NAND4/2, NAND2/2
  In1/1 -> NAND6/2, NAND5/2, NAND3/2, NAND3/1
  In2/1 -> NAND6/1, NAND4/1, NAND/2, NAND/1
  In4/1 -> NAND4/3
  In3/1 -> NAND2/3
  NAND/1 -> NAND5/1, NAND2/1
  NAND1/1 -> Out1/1
  In6/1 -> NAND6/3
  NAND5/1 -> NAND1/3
  NAND4/1 -> NAND1/2
  In7/1 -> NAND2/4, NAND4/4, NAND5/4, NAND6/4
  NAND2/1 -> NAND1/1

== system cpu_von_nuemann/CPU/ALU/Subsystem7/Subsystem2/Subsystem4/Subsystem ==
  In1 : Inport
  In2 : Inport  Port=2
  In3 : Inport  Port=3
  In4 : Inport  Port=4
  In5 : Inport  Port=5
  In6 : Inport  Port=6
  In7 : Inport  Port=7
  NAND : Logic  Operator=NAND  AllPortsSameDT=off  OutDataTypeStr=boolean
  NAND{1..2,4..6} (5 alike) : Logic  Operator=NAND  Inputs=4  AllPortsSameDT=off  OutDataTypeStr=boolean
  NAND3 : Logic  Operator=NAND  AllPortsSameDT=off  OutDataTypeStr=boolean
  Out1 : Outport
  wires:
  NAND6/1 -> NAND1/4
  In5/1 -> NAND5/3
  NAND3/1 -> NAND4/2, NAND2/2
  In1/1 -> NAND6/2, NAND5/2, NAND3/2, NAND3/1
  In2/1 -> NAND6/1, NAND4/1, NAND/2, NAND/1
  In4/1 -> NAND4/3
  In3/1 -> NAND2/3
  NAND/1 -> NAND5/1, NAND2/1
  NAND1/1 -> Out1/1
  In6/1 -> NAND6/3
  NAND5/1 -> NAND1/3
  NAND4/1 -> NAND1/2
  In7/1 -> NAND2/4, NAND4/4, NAND5/4, NAND6/4
  NAND2/1 -> NAND1/1

== system cpu_von_nuemann/CPU/ALU/Subsystem7/Subsystem2/Subsystem4/Subsystem1 ==
  In1 : Inport
  In2 : Inport  Port=2
  In3 : Inport  Port=3
  In4 : Inport  Port=4
  In5 : Inport  Port=5
  In6 : Inport  Port=6
  In7 : Inport  Port=7
  NAND : Logic  Operator=NAND  AllPortsSameDT=off  OutDataTypeStr=boolean
  NAND{1..2,4..6} (5 alike) : Logic  Operator=NAND  Inputs=4  AllPortsSameDT=off  OutDataTypeStr=boolean
  NAND3 : Logic  Operator=NAND  AllPortsSameDT=off  OutDataTypeStr=boolean
  Out1 : Outport
  wires:
  NAND6/1 -> NAND1/4
  In5/1 -> NAND5/3
  NAND3/1 -> NAND4/2, NAND2/2
  In1/1 -> NAND6/2, NAND5/2, NAND3/2, NAND3/1
  In2/1 -> NAND6/1, NAND4/1, NAND/2, NAND/1
  In4/1 -> NAND4/3
  In3/1 -> NAND2/3
  NAND/1 -> NAND5/1, NAND2/1
  NAND1/1 -> Out1/1
  In6/1 -> NAND6/3
  NAND5/1 -> NAND1/3
  NAND4/1 -> NAND1/2
  In7/1 -> NAND2/4, NAND4/4, NAND5/4, NAND6/4
  NAND2/1 -> NAND1/1

== system cpu_von_nuemann/CPU/ALU/Subsystem7/Subsystem2/Subsystem4/Subsystem2 ==
  In1 : Inport
  In2 : Inport  Port=2
  In3 : Inport  Port=3
  In4 : Inport  Port=4
  In5 : Inport  Port=5
  In6 : Inport  Port=6
  In7 : Inport  Port=7
  NAND : Logic  Operator=NAND  AllPortsSameDT=off  OutDataTypeStr=boolean
  NAND{1..2,4..6} (5 alike) : Logic  Operator=NAND  Inputs=4  AllPortsSameDT=off  OutDataTypeStr=boolean
  NAND3 : Logic  Operator=NAND  AllPortsSameDT=off  OutDataTypeStr=boolean
  Out1 : Outport
  wires:
  NAND6/1 -> NAND1/4
  In5/1 -> NAND5/3
  NAND3/1 -> NAND4/2, NAND2/2
  In1/1 -> NAND6/2, NAND5/2, NAND3/2, NAND3/1
  In2/1 -> NAND6/1, NAND4/1, NAND/2, NAND/1
  In4/1 -> NAND4/3
  In3/1 -> NAND2/3
  NAND/1 -> NAND5/1, NAND2/1
  NAND1/1 -> Out1/1
  In6/1 -> NAND6/3
  NAND5/1 -> NAND1/3
  NAND4/1 -> NAND1/2
  In7/1 -> NAND2/4, NAND4/4, NAND5/4, NAND6/4
  NAND2/1 -> NAND1/1

== system cpu_von_nuemann/CPU/ALU/Subsystem7/Subsystem2/Subsystem4/Subsystem3 ==
  In1 : Inport
  In2 : Inport  Port=2
  In3 : Inport  Port=3
  In4 : Inport  Port=4
  In5 : Inport  Port=5
  In6 : Inport  Port=6
  In7 : Inport  Port=7
  NAND : Logic  Operator=NAND  AllPortsSameDT=off  OutDataTypeStr=boolean
  NAND{1..2,4..6} (5 alike) : Logic  Operator=NAND  Inputs=4  AllPortsSameDT=off  OutDataTypeStr=boolean
  NAND3 : Logic  Operator=NAND  AllPortsSameDT=off  OutDataTypeStr=boolean
  Out1 : Outport
  wires:
  NAND6/1 -> NAND1/4
  In5/1 -> NAND5/3
  NAND3/1 -> NAND4/2, NAND2/2
  In1/1 -> NAND6/2, NAND5/2, NAND3/2, NAND3/1
  In2/1 -> NAND6/1, NAND4/1, NAND/2, NAND/1
  In4/1 -> NAND4/3
  In3/1 -> NAND2/3
  NAND/1 -> NAND5/1, NAND2/1
  NAND1/1 -> Out1/1
  In6/1 -> NAND6/3
  NAND5/1 -> NAND1/3
  NAND4/1 -> NAND1/2
  In7/1 -> NAND2/4, NAND4/4, NAND5/4, NAND6/4
  NAND2/1 -> NAND1/1

== system cpu_von_nuemann/CPU/ALU/Subsystem7/Subsystem2/Subsystem4/Subsystem4 ==
  In1 : Inport
  In2 : Inport  Port=2
  In3 : Inport  Port=3
  In4 : Inport  Port=4
  In5 : Inport  Port=5
  In6 : Inport  Port=6
  In7 : Inport  Port=7
  NAND : Logic  Operator=NAND  AllPortsSameDT=off  OutDataTypeStr=boolean
  NAND{1..2,4..6} (5 alike) : Logic  Operator=NAND  Inputs=4  AllPortsSameDT=off  OutDataTypeStr=boolean
  NAND3 : Logic  Operator=NAND  AllPortsSameDT=off  OutDataTypeStr=boolean
  Out1 : Outport
  wires:
  NAND6/1 -> NAND1/4
  In5/1 -> NAND5/3
  NAND3/1 -> NAND4/2, NAND2/2
  In1/1 -> NAND6/2, NAND5/2, NAND3/2, NAND3/1
  In2/1 -> NAND6/1, NAND4/1, NAND/2, NAND/1
  In4/1 -> NAND4/3
  In3/1 -> NAND2/3
  NAND/1 -> NAND5/1, NAND2/1
  NAND1/1 -> Out1/1
  In6/1 -> NAND6/3
  NAND5/1 -> NAND1/3
  NAND4/1 -> NAND1/2
  In7/1 -> NAND2/4, NAND4/4, NAND5/4, NAND6/4
  NAND2/1 -> NAND1/1

== system cpu_von_nuemann/CPU/ALU/Subsystem7/Subsystem2/Subsystem4/Subsystem5 ==
  In1 : Inport
  In2 : Inport  Port=2
  In3 : Inport  Port=3
  In4 : Inport  Port=4
  In5 : Inport  Port=5
  In6 : Inport  Port=6
  In7 : Inport  Port=7
  NAND : Logic  Operator=NAND  AllPortsSameDT=off  OutDataTypeStr=boolean
  NAND{1..2,4..6} (5 alike) : Logic  Operator=NAND  Inputs=4  AllPortsSameDT=off  OutDataTypeStr=boolean
  NAND3 : Logic  Operator=NAND  AllPortsSameDT=off  OutDataTypeStr=boolean
  Out1 : Outport
  wires:
  NAND6/1 -> NAND1/4
  In5/1 -> NAND5/3
  NAND3/1 -> NAND4/2, NAND2/2
  In1/1 -> NAND6/2, NAND5/2, NAND3/2, NAND3/1
  In2/1 -> NAND6/1, NAND4/1, NAND/2, NAND/1
  In4/1 -> NAND4/3
  In3/1 -> NAND2/3
  NAND/1 -> NAND5/1, NAND2/1
  NAND1/1 -> Out1/1
  In6/1 -> NAND6/3
  NAND5/1 -> NAND1/3
  NAND4/1 -> NAND1/2
  In7/1 -> NAND2/4, NAND4/4, NAND5/4, NAND6/4
  NAND2/1 -> NAND1/1

== system cpu_von_nuemann/CPU/ALU/Subsystem7/Subsystem2/Subsystem4/Subsystem6 ==
  In1 : Inport
  In2 : Inport  Port=2
  In3 : Inport  Port=3
  In4 : Inport  Port=4
  In5 : Inport  Port=5
  In6 : Inport  Port=6
  In7 : Inport  Port=7
  NAND : Logic  Operator=NAND  AllPortsSameDT=off  OutDataTypeStr=boolean
  NAND{1..2,4..6} (5 alike) : Logic  Operator=NAND  Inputs=4  AllPortsSameDT=off  OutDataTypeStr=boolean
  NAND3 : Logic  Operator=NAND  AllPortsSameDT=off  OutDataTypeStr=boolean
  Out1 : Outport
  wires:
  NAND6/1 -> NAND1/4
  In5/1 -> NAND5/3
  NAND3/1 -> NAND4/2, NAND2/2
  In1/1 -> NAND6/2, NAND5/2, NAND3/2, NAND3/1
  In2/1 -> NAND6/1, NAND4/1, NAND/2, NAND/1
  In4/1 -> NAND4/3
  In3/1 -> NAND2/3
  NAND/1 -> NAND5/1, NAND2/1
  NAND1/1 -> Out1/1
  In6/1 -> NAND6/3
  NAND5/1 -> NAND1/3
  NAND4/1 -> NAND1/2
  In7/1 -> NAND2/4, NAND4/4, NAND5/4, NAND6/4
  NAND2/1 -> NAND1/1

== system cpu_von_nuemann/CPU/ALU/Subsystem7/Subsystem2/Subsystem4/Subsystem7 ==
  In1 : Inport
  In2 : Inport  Port=2
  In3 : Inport  Port=3
  In4 : Inport  Port=4
  In5 : Inport  Port=5
  In6 : Inport  Port=6
  In7 : Inport  Port=7
  NAND : Logic  Operator=NAND  AllPortsSameDT=off  OutDataTypeStr=boolean
  NAND{1..2,4..6} (5 alike) : Logic  Operator=NAND  Inputs=4  AllPortsSameDT=off  OutDataTypeStr=boolean
  NAND3 : Logic  Operator=NAND  AllPortsSameDT=off  OutDataTypeStr=boolean
  Out1 : Outport
  wires:
  NAND6/1 -> NAND1/4
  In5/1 -> NAND5/3
  NAND3/1 -> NAND4/2, NAND2/2
  In1/1 -> NAND6/2, NAND5/2, NAND3/2, NAND3/1
  In2/1 -> NAND6/1, NAND4/1, NAND/2, NAND/1
  In4/1 -> NAND4/3
  In3/1 -> NAND2/3
  NAND/1 -> NAND5/1, NAND2/1
  NAND1/1 -> Out1/1
  In6/1 -> NAND6/3
  NAND5/1 -> NAND1/3
  NAND4/1 -> NAND1/2
  In7/1 -> NAND2/4, NAND4/4, NAND5/4, NAND6/4
  NAND2/1 -> NAND1/1

== system cpu_von_nuemann/CPU/ALU/Subsystem7/Subsystem2/Subsystem5/Subsystem ==
  In1 : Inport
  In2 : Inport  Port=2
  In3 : Inport  Port=3
  In4 : Inport  Port=4
  In5 : Inport  Port=5
  In6 : Inport  Port=6
  In7 : Inport  Port=7
  NAND : Logic  Operator=NAND  AllPortsSameDT=off  OutDataTypeStr=boolean
  NAND{1..2,4..6} (5 alike) : Logic  Operator=NAND  Inputs=4  AllPortsSameDT=off  OutDataTypeStr=boolean
  NAND3 : Logic  Operator=NAND  AllPortsSameDT=off  OutDataTypeStr=boolean
  Out1 : Outport
  wires:
  NAND6/1 -> NAND1/4
  In5/1 -> NAND5/3
  NAND3/1 -> NAND4/2, NAND2/2
  In1/1 -> NAND6/2, NAND5/2, NAND3/2, NAND3/1
  In2/1 -> NAND6/1, NAND4/1, NAND/2, NAND/1
  In4/1 -> NAND4/3
  In3/1 -> NAND2/3
  NAND/1 -> NAND5/1, NAND2/1
  NAND1/1 -> Out1/1
  In6/1 -> NAND6/3
  NAND5/1 -> NAND1/3
  NAND4/1 -> NAND1/2
  In7/1 -> NAND2/4, NAND4/4, NAND5/4, NAND6/4
  NAND2/1 -> NAND1/1

== system cpu_von_nuemann/CPU/ALU/Subsystem7/Subsystem2/Subsystem5/Subsystem1 ==
  In1 : Inport
  In2 : Inport  Port=2
  In3 : Inport  Port=3
  In4 : Inport  Port=4
  In5 : Inport  Port=5
  In6 : Inport  Port=6
  In7 : Inport  Port=7
  NAND : Logic  Operator=NAND  AllPortsSameDT=off  OutDataTypeStr=boolean
  NAND{1..2,4..6} (5 alike) : Logic  Operator=NAND  Inputs=4  AllPortsSameDT=off  OutDataTypeStr=boolean
  NAND3 : Logic  Operator=NAND  AllPortsSameDT=off  OutDataTypeStr=boolean
  Out1 : Outport
  wires:
  NAND6/1 -> NAND1/4
  In5/1 -> NAND5/3
  NAND3/1 -> NAND4/2, NAND2/2
  In1/1 -> NAND6/2, NAND5/2, NAND3/2, NAND3/1
  In2/1 -> NAND6/1, NAND4/1, NAND/2, NAND/1
  In4/1 -> NAND4/3
  In3/1 -> NAND2/3
  NAND/1 -> NAND5/1, NAND2/1
  NAND1/1 -> Out1/1
  In6/1 -> NAND6/3
  NAND5/1 -> NAND1/3
  NAND4/1 -> NAND1/2
  In7/1 -> NAND2/4, NAND4/4, NAND5/4, NAND6/4
  NAND2/1 -> NAND1/1

== system cpu_von_nuemann/CPU/ALU/Subsystem7/Subsystem2/Subsystem5/Subsystem2 ==
  In1 : Inport
  In2 : Inport  Port=2
  In3 : Inport  Port=3
  In4 : Inport  Port=4
  In5 : Inport  Port=5
  In6 : Inport  Port=6
  In7 : Inport  Port=7
  NAND : Logic  Operator=NAND  AllPortsSameDT=off  OutDataTypeStr=boolean
  NAND{1..2,4..6} (5 alike) : Logic  Operator=NAND  Inputs=4  AllPortsSameDT=off  OutDataTypeStr=boolean
  NAND3 : Logic  Operator=NAND  AllPortsSameDT=off  OutDataTypeStr=boolean
  Out1 : Outport
  wires:
  NAND6/1 -> NAND1/4
  In5/1 -> NAND5/3
  NAND3/1 -> NAND4/2, NAND2/2
  In1/1 -> NAND6/2, NAND5/2, NAND3/2, NAND3/1
  In2/1 -> NAND6/1, NAND4/1, NAND/2, NAND/1
  In4/1 -> NAND4/3
  In3/1 -> NAND2/3
  NAND/1 -> NAND5/1, NAND2/1
  NAND1/1 -> Out1/1
  In6/1 -> NAND6/3
  NAND5/1 -> NAND1/3
  NAND4/1 -> NAND1/2
  In7/1 -> NAND2/4, NAND4/4, NAND5/4, NAND6/4
  NAND2/1 -> NAND1/1

== system cpu_von_nuemann/CPU/ALU/Subsystem7/Subsystem2/Subsystem5/Subsystem3 ==
  In1 : Inport
  In2 : Inport  Port=2
  In3 : Inport  Port=3
  In4 : Inport  Port=4
  In5 : Inport  Port=5
  In6 : Inport  Port=6
  In7 : Inport  Port=7
  NAND : Logic  Operator=NAND  AllPortsSameDT=off  OutDataTypeStr=boolean
  NAND{1..2,4..6} (5 alike) : Logic  Operator=NAND  Inputs=4  AllPortsSameDT=off  OutDataTypeStr=boolean
  NAND3 : Logic  Operator=NAND  AllPortsSameDT=off  OutDataTypeStr=boolean
  Out1 : Outport
  wires:
  NAND6/1 -> NAND1/4
  In5/1 -> NAND5/3
  NAND3/1 -> NAND4/2, NAND2/2
  In1/1 -> NAND6/2, NAND5/2, NAND3/2, NAND3/1
  In2/1 -> NAND6/1, NAND4/1, NAND/2, NAND/1
  In4/1 -> NAND4/3
  In3/1 -> NAND2/3
  NAND/1 -> NAND5/1, NAND2/1
  NAND1/1 -> Out1/1
  In6/1 -> NAND6/3
  NAND5/1 -> NAND1/3
  NAND4/1 -> NAND1/2
  In7/1 -> NAND2/4, NAND4/4, NAND5/4, NAND6/4
  NAND2/1 -> NAND1/1

== system cpu_von_nuemann/CPU/ALU/Subsystem7/Subsystem2/Subsystem5/Subsystem4 ==
  In1 : Inport
  In2 : Inport  Port=2
  In3 : Inport  Port=3
  In4 : Inport  Port=4
  In5 : Inport  Port=5
  In6 : Inport  Port=6
  In7 : Inport  Port=7
  NAND : Logic  Operator=NAND  AllPortsSameDT=off  OutDataTypeStr=boolean
  NAND{1..2,4..6} (5 alike) : Logic  Operator=NAND  Inputs=4  AllPortsSameDT=off  OutDataTypeStr=boolean
  NAND3 : Logic  Operator=NAND  AllPortsSameDT=off  OutDataTypeStr=boolean
  Out1 : Outport
  wires:
  NAND6/1 -> NAND1/4
  In5/1 -> NAND5/3
  NAND3/1 -> NAND4/2, NAND2/2
  In1/1 -> NAND6/2, NAND5/2, NAND3/2, NAND3/1
  In2/1 -> NAND6/1, NAND4/1, NAND/2, NAND/1
  In4/1 -> NAND4/3
  In3/1 -> NAND2/3
  NAND/1 -> NAND5/1, NAND2/1
  NAND1/1 -> Out1/1
  In6/1 -> NAND6/3
  NAND5/1 -> NAND1/3
  NAND4/1 -> NAND1/2
  In7/1 -> NAND2/4, NAND4/4, NAND5/4, NAND6/4
  NAND2/1 -> NAND1/1

== system cpu_von_nuemann/CPU/ALU/Subsystem7/Subsystem2/Subsystem5/Subsystem5 ==
  In1 : Inport
  In2 : Inport  Port=2
  In3 : Inport  Port=3
  In4 : Inport  Port=4
  In5 : Inport  Port=5
  In6 : Inport  Port=6
  In7 : Inport  Port=7
  NAND : Logic  Operator=NAND  AllPortsSameDT=off  OutDataTypeStr=boolean
  NAND{1..2,4..6} (5 alike) : Logic  Operator=NAND  Inputs=4  AllPortsSameDT=off  OutDataTypeStr=boolean
  NAND3 : Logic  Operator=NAND  AllPortsSameDT=off  OutDataTypeStr=boolean
  Out1 : Outport
  wires:
  NAND6/1 -> NAND1/4
  In5/1 -> NAND5/3
  NAND3/1 -> NAND4/2, NAND2/2
  In1/1 -> NAND6/2, NAND5/2, NAND3/2, NAND3/1
  In2/1 -> NAND6/1, NAND4/1, NAND/2, NAND/1
  In4/1 -> NAND4/3
  In3/1 -> NAND2/3
  NAND/1 -> NAND5/1, NAND2/1
  NAND1/1 -> Out1/1
  In6/1 -> NAND6/3
  NAND5/1 -> NAND1/3
  NAND4/1 -> NAND1/2
  In7/1 -> NAND2/4, NAND4/4, NAND5/4, NAND6/4
  NAND2/1 -> NAND1/1

== system cpu_von_nuemann/CPU/ALU/Subsystem7/Subsystem2/Subsystem5/Subsystem6 ==
  In1 : Inport
  In2 : Inport  Port=2
  In3 : Inport  Port=3
  In4 : Inport  Port=4
  In5 : Inport  Port=5
  In6 : Inport  Port=6
  In7 : Inport  Port=7
  NAND : Logic  Operator=NAND  AllPortsSameDT=off  OutDataTypeStr=boolean
  NAND{1..2,4..6} (5 alike) : Logic  Operator=NAND  Inputs=4  AllPortsSameDT=off  OutDataTypeStr=boolean
  NAND3 : Logic  Operator=NAND  AllPortsSameDT=off  OutDataTypeStr=boolean
  Out1 : Outport
  wires:
  NAND6/1 -> NAND1/4
  In5/1 -> NAND5/3
  NAND3/1 -> NAND4/2, NAND2/2
  In1/1 -> NAND6/2, NAND5/2, NAND3/2, NAND3/1
  In2/1 -> NAND6/1, NAND4/1, NAND/2, NAND/1
  In4/1 -> NAND4/3
  In3/1 -> NAND2/3
  NAND/1 -> NAND5/1, NAND2/1
  NAND1/1 -> Out1/1
  In6/1 -> NAND6/3
  NAND5/1 -> NAND1/3
  NAND4/1 -> NAND1/2
  In7/1 -> NAND2/4, NAND4/4, NAND5/4, NAND6/4
  NAND2/1 -> NAND1/1

== system cpu_von_nuemann/CPU/ALU/Subsystem7/Subsystem2/Subsystem5/Subsystem7 ==
  In1 : Inport
  In2 : Inport  Port=2
  In3 : Inport  Port=3
  In4 : Inport  Port=4
  In5 : Inport  Port=5
  In6 : Inport  Port=6
  In7 : Inport  Port=7
  NAND : Logic  Operator=NAND  AllPortsSameDT=off  OutDataTypeStr=boolean
  NAND{1..2,4..6} (5 alike) : Logic  Operator=NAND  Inputs=4  AllPortsSameDT=off  OutDataTypeStr=boolean
  NAND3 : Logic  Operator=NAND  AllPortsSameDT=off  OutDataTypeStr=boolean
  Out1 : Outport
  wires:
  NAND6/1 -> NAND1/4
  In5/1 -> NAND5/3
  NAND3/1 -> NAND4/2, NAND2/2
  In1/1 -> NAND6/2, NAND5/2, NAND3/2, NAND3/1
  In2/1 -> NAND6/1, NAND4/1, NAND/2, NAND/1
  In4/1 -> NAND4/3
  In3/1 -> NAND2/3
  NAND/1 -> NAND5/1, NAND2/1
  NAND1/1 -> Out1/1
  In6/1 -> NAND6/3
  NAND5/1 -> NAND1/3
  NAND4/1 -> NAND1/2
  In7/1 -> NAND2/4, NAND4/4, NAND5/4, NAND6/4
  NAND2/1 -> NAND1/1
